simulink model "Bicycle_model"  (R2025b)
settings: Solver=FixedStepAuto  StartTime=0.0  StopTime=20  FixedStep=1/200  RelTol=1e-3
libraries: autolibshared x1
settings Model: Creator=noahstairs  LastModifiedBy=noahstairs

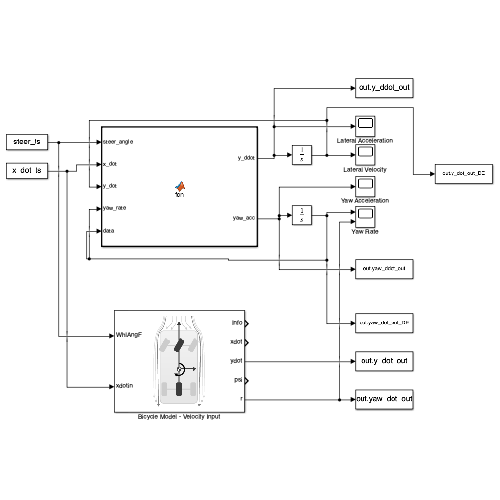
[thumbnail: Simulink's stored preview of the top-level diagram]
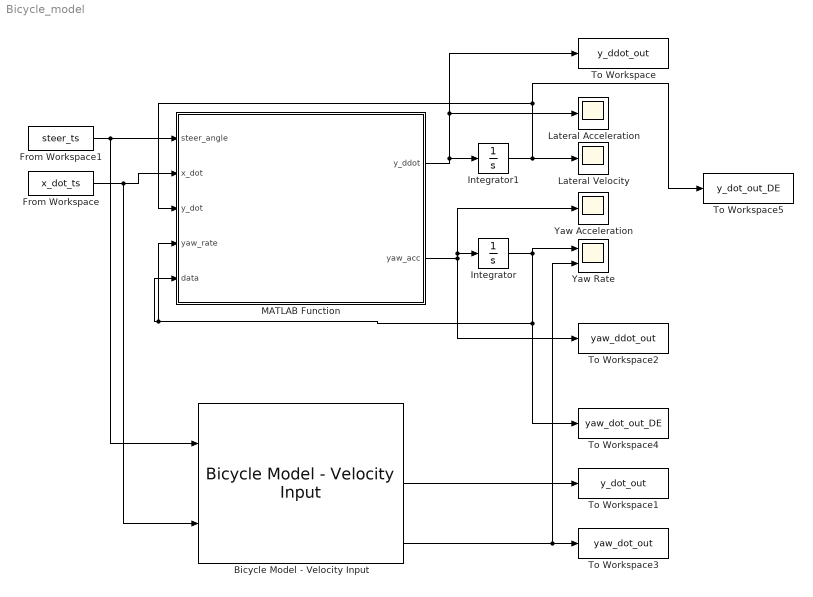
== system Bicycle_model ==
  Bicycle Model - Velocity Input : autolibshared/Bicycle Model - Velocity Input  trackMode=Single (bicycle)  inputMode=External longitudinal velocity  frontSteerMode=on  rearSteerMode=off  windMode=off  muMode=off  extFMode=off  extMMode=off  aMode=3  NF=2  NR=2  m=2000  a=1.4  b=1.6  h=0.35  X_o=0  xdot_o=0  CalphaMode=off  sigmaMode=on  w=[1.4,1.4]  Cy_f=12000  Cy_r=11000  sigma_f=.1  sigma_r=.1  alpha_f_brk=[-.1 .1]  Cy_f_data=[-9e3 9e3]  alpha_r_brk=[-.1 .1]  Cy_r_data=[-9e3 9e3]  Y_o=0  ydot_o=0  Izz=4000  psi_o=0  r_o=0  Af=2  Cd=.3  Cl=.1  Cpm=.1  beta_w=[0 0.01:0.01:0.3]  Cs=[0 0.01:0.01:0.3]  Cym=[0 1e-6:0.01:0.3]  Pabs=101325  Tair=273  g=9.81  mu=1  xdot_tol=.01  Fznom=5000  Fxtire_sat=1e6  Fytire_sat=1e6  longOff=0  latOff=0  vertOff=0
      settings: LibrarySourceBlock=drivingscenarioandsensors/Bicycle Model - Velocity Input
  From Workspace : FromWorkspace  VariableName=x_dot_ts  SampleTime=-1
  From Workspace1 : FromWorkspace  VariableName=steer_ts  SampleTime=-1
  Integrator : Integrator
  Integrator1 : Integrator
  Lateral Acceleration : Scope
      settings: ActiveDisplayYMinimum=-1  ActiveDisplayYMaximum=1  DataLoggingVariableName=ScopeData2
  Lateral Velocity : Scope
      settings: ActiveDisplayYMinimum=-1  ActiveDisplayYMaximum=1
  MATLAB Function : MATLAB Function  TreatAsAtomicUnit=on
  To Workspace : ToWorkspace  VariableName=y_ddot_out  SaveFormat=Timeseries  SampleTime=-1
  To Workspace1 : ToWorkspace  VariableName=y_dot_out  SaveFormat=Timeseries  SampleTime=-1
  To Workspace2 : ToWorkspace  VariableName=yaw_ddot_out  SaveFormat=Timeseries  SampleTime=-1
  To Workspace3 : ToWorkspace  VariableName=yaw_dot_out  SaveFormat=Timeseries  SampleTime=-1
  To Workspace4 : ToWorkspace  VariableName=yaw_dot_out_DE  SaveFormat=Timeseries  SampleTime=-1
  To Workspace5 : ToWorkspace  VariableName=y_dot_out_DE  SaveFormat=Timeseries  SampleTime=-1
  Yaw Acceleration : Scope
      settings: ActiveDisplayYMinimum=-1  ActiveDisplayYMaximum=1  DataLoggingVariableName=ScopeData3
  Yaw Rate : Scope  NumInputPorts=2
      settings: ActiveDisplayYMinimum=-1  ActiveDisplayYMaximum=1
  wires:
  From Workspace1/1 -> Bicycle Model - Velocity Input/1, MATLAB Function/1(steer_angle)
  From Workspace/1 -> Bicycle Model - Velocity Input/2, MATLAB Function/2(x_dot)
  MATLAB Function/2(yaw_acc) -> Yaw Acceleration/1, Integrator/1, To Workspace2/1
  MATLAB Function/1(y_ddot) -> To Workspace/1, Lateral Acceleration/1, Integrator1/1
  Integrator1/1 -> To Workspace5/1, MATLAB Function/3(y_dot), Lateral Velocity/1
  Integrator/1 -> To Workspace4/1, MATLAB Function/5(data), MATLAB Function/4(yaw_rate), Yaw Rate/1
  Bicycle Model - Velocity Input/5 -> Yaw Rate/2, To Workspace3/1
  Bicycle Model - Velocity Input/3 -> To Workspace1/1

== matlab function Bicycle_model/MATLAB Function ==
  data: steer_angle input; y_ddot output; x_dot input; y_dot input; yaw_rate input; yaw_acc output; data input
function [y_ddot, yaw_acc] = fcn(steer_angle, x_dot, y_dot, yaw_rate, data)

% Vehicle Parameters
m = 2000; % kg
Iz = 4000; % kg m^2
L1 = 1.4; % m
L2 = 1.6; % m
Cf = 12e3; % N/rad
Cr = 11e3; % N/rad

% A
A = [-(2*Cf+2*Cr)/(m*x_dot), (2*Cr*L2-2*Cf*L1)/(m*x_dot)-x_dot ;
      (2*Cr*L2-2*Cf*L1)/(Iz*x_dot), -(2*Cf*L1^2+2*Cr*L2^2)/(Iz*x_dot)];
   
% B
B = [2*Cf/m ; 2*Cf*L1/Iz];

%X_Dot
X = [y_dot ; yaw_rate];
X_Dot = A*X + B*steer_angle;

y_ddot = X_Dot(1);
yaw_acc = X_Dot(2);
